simulink model "test_dropout"  (R2017a)
settings: Solver=FixedStepDiscrete  StartTime=0.0  StopTime=10.0  RelTol=1e-3
undefined symbols (not defined in the file or in its folder): gray
libraries: ad_blocks x1, visionsources x1, visiongeotforms x1
settings Model: Creator=eruffaldi  LastModifiedBy=eruffaldi

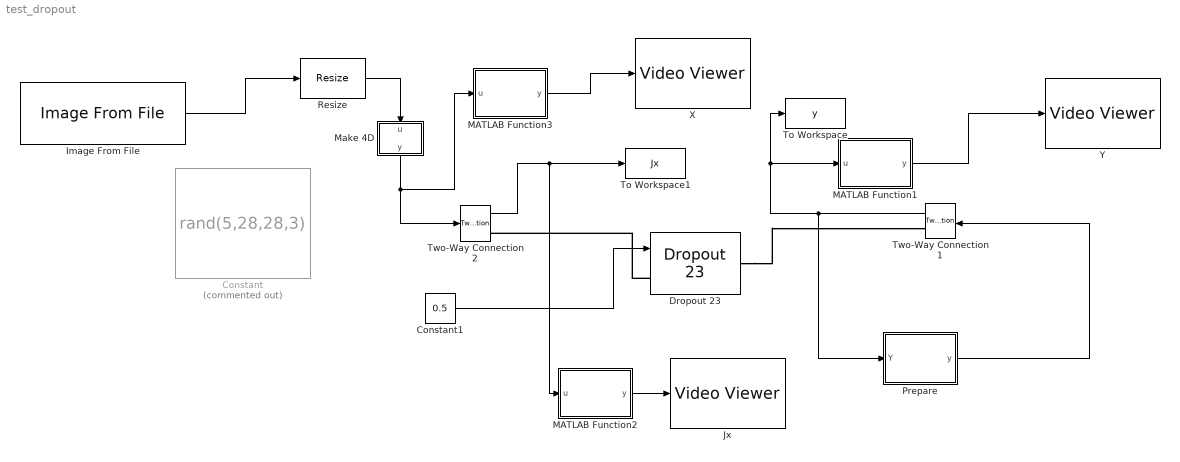
== system test_dropout ==
  Constant : Constant  Commented=on  Value=rand(5,28,28,3)
  Constant1 : Constant  Value=0.5
  Dropout 23 : ad_blocks/Dropout 23
  Image From File : visionsources/Image From File  Tag=vipblks_nd  FileName=peppers.png  imagePorts=One multidimensional signal  Ts=inf  ImageDataType=double  Signed=on  WordLength=16  sdImageDataType=uint(8)  FractionLengthMode=User-defined  FractionLength=15  OutPortLabels=R|G|B
      settings: SourceProductName=Computer Vision System Toolbox
  Jx : VideoViewer  colormapValue=gray(256)  FigPos=[1 894 1440 774]
  MATLAB Function1 : MATLAB Function  TreatAsAtomicUnit=on
  MATLAB Function2 : MATLAB Function  TreatAsAtomicUnit=on
  MATLAB Function3 : MATLAB Function  TreatAsAtomicUnit=on
  Make 4D : MATLAB Function  TreatAsAtomicUnit=on
  "Prepare " : MATLAB Function  TreatAsAtomicUnit=on
  Resize : visiongeotforms/Resize  specify=Number of output columns and preserve aspect ratio  rfactor=[200 150]  outCols=200  outRows=25  outRowsCols=[25 35]  interp_method=Bilinear  antialias=on  useROI=off  roiFlag=off  prodOutputMode=Binary point scaling  prodOutputWordLength=32  prodOutputFracLength=10  roundingMode=Nearest  overflowMode=on
      settings: SourceProductName=Computer Vision System Toolbox  SourceProductBaseCode=VP
  To Workspace : ToWorkspace  VariableName=y  SaveFormat=Timeseries  SampleTime=-1
  To Workspace1 : ToWorkspace  VariableName=Jx  SaveFormat=Timeseries  SampleTime=-1
  Two-Way Connection1 : TwoWayConnection
  Two-Way Connection2 : TwoWayConnection
  X : VideoViewer  colormapValue=gray(256)  FigPos=[270 851 418 304]
  Y : VideoViewer  colormapValue=gray(256)  FigPos=[1 894 1440 774]
  wires:
  "Prepare "/1(y) -> Two-Way Connection1/1
  Resize/1 -> Make 4D/1(u)
  Two-Way Connection1/1 -> "Prepare "/1(Y), MATLAB Function1/1(u), To Workspace/1
  Image From File/1 -> Resize/1
  Make 4D/1(y) -> MATLAB Function3/1(u), Two-Way Connection2/1
  Two-Way Connection2/1 -> MATLAB Function2/1(u), To Workspace1/1
  MATLAB Function1/1(y) -> Y/1
  MATLAB Function3/1(y) -> X/1
  MATLAB Function2/1(y) -> Jx/1
  Constant1/1 -> Dropout 23/1
  connections:
  Dropout 23/LConn1 -- Two-Way Connection2/RConn1
  Dropout 23/RConn1 -- Two-Way Connection1/RConn1

== matlab function test_dropout/MATLAB Function1 ==
  data: y output; u input
function y = fcn(u)
y = squeeze(u(1,:,:,:));

== matlab function test_dropout/Prepare  ==
  data: y output; Y input
function y = fcn(Y)

y = ones(size(Y),'like',Y);

== matlab function test_dropout/MATLAB Function2 ==
  data: y output; u input
function y = fcn(u)
y = squeeze(u(1,:,:,:));

== matlab function test_dropout/MATLAB Function3 ==
  data: y output; u input
function y = fcn(u)
y = squeeze(u(1,:,:,:));

== matlab function test_dropout/Make 4D ==
  data: y output; u input
function y = fcn(u)
y = reshape(u,[1,size(u)]);
